simulink model "Stage_3_Multi_ECU_CAN_Network"  (R2025a)
settings: Solver=VariableStepAuto  StartTime=0.0  StopTime=10.0  RelTol=1e-3
libraries: SignalEditorBlockLib x13, canmsglib x8, simulink x1
settings Model: Creator=sitam  LastModifiedBy=sitam

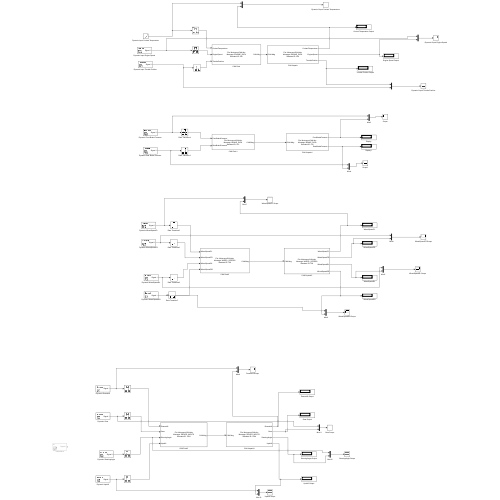
[thumbnail: Simulink's stored preview of the top-level diagram]
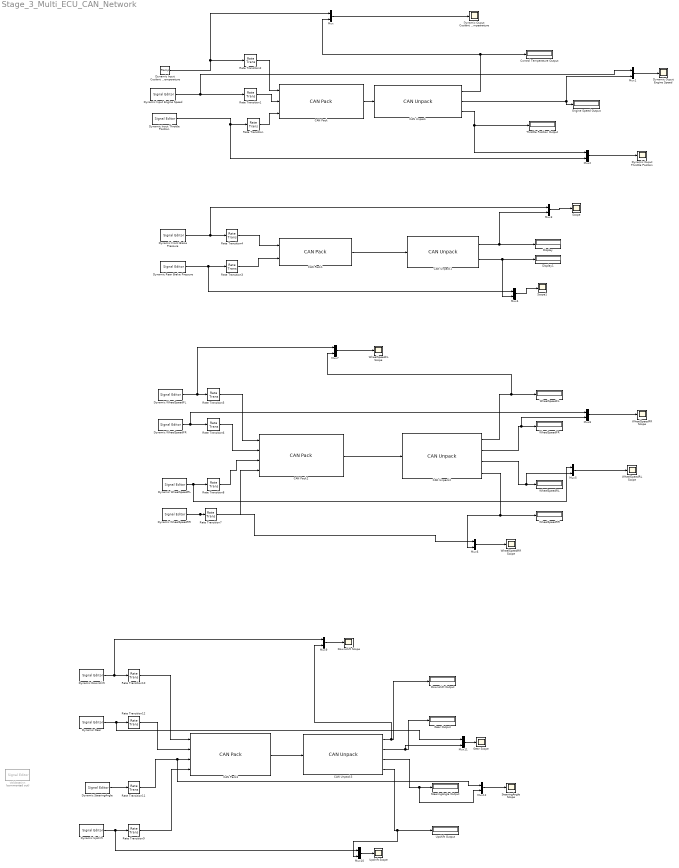
== system Stage_3_Multi_ECU_CAN_Network ==
  CAN Pack : canmsglib/CAN Pack  CANdbFile=C:\Users\sitam\OneDrive\Projects\CAN Bus Project\MotorsportCAN.dbc  MsgList=ENGINE_DATA  MsgName=ENGINE_DATA  MsgIDType=Standard (11-bit identifier)  MsgIdentifier=256  CANIDInput=off  MsgLength=8  Remote=off  ApplyMinMax=off  BusOutput=off  SignalInfo={'CoolantTemperature','24','8','LE','unsigned','Standard','0','1','-40','-40','150';'EngineSpeed','0','16','LE','unsigned','Standard','0','0.25','0','0','15000';'ThrottlePosition','16','8','LE','unsigned','Standard','0','0.4','0','0','100'}
      settings: LibrarySourceBlock=canlib/CAN Pack  DataFormat=CANdb specified signals
  CAN Pack1 : canmsglib/CAN Pack  CANdbFile=C:\Users\sitam\OneDrive\Projects\CAN Bus Project\MotorsportCAN.dbc  MsgList=BRAKE_DATA  MsgName=BRAKE_DATA  MsgIDType=Standard (11-bit identifier)  MsgIdentifier=512  CANIDInput=off  MsgLength=8  Remote=off  ApplyMinMax=off  BusOutput=off  SignalInfo={'FrontBrakePressure','0','16','LE','unsigned','Standard','0','0.01','0','0','200';'RearBrakePressure','16','16','LE','unsigned','Standard','0','0.01','0','0','200'}
      settings: LibrarySourceBlock=canlib/CAN Pack  DataFormat=CANdb specified signals
  CAN Pack2 : canmsglib/CAN Pack  CANdbFile=C:\Users\sitam\OneDrive\Projects\CAN Bus Project\MotorsportCAN.dbc  MsgList=WHEEL_SPEEDS  MsgName=WHEEL_SPEEDS  MsgIDType=Standard (11-bit identifier)  MsgIdentifier=768  CANIDInput=off  MsgLength=8  Remote=off  ApplyMinMax=off  BusOutput=off  SignalInfo={'WheelSpeedFL','0','16','LE','unsigned','Standard','0','0.01','0','0','350';'WheelSpeedFR','16','16','LE','unsigned','Standard','0','0.01','0','0','350';'WheelSpeedRL','32','16','LE','unsigned','Standard','0','0.01','0','0','350';'WheelSpeedRR','48','16','LE','unsigned','Standard','0','0.01','0','0','350'}
      settings: LibrarySourceBlock=canlib/CAN Pack  DataFormat=CANdb specified signals
  CAN Pack3 : canmsglib/CAN Pack  CANdbFile=C:\Users\sitam\OneDrive\Projects\CAN Bus Project\MotorsportCAN.dbc  MsgList=DRIVER_INPUTS  MsgName=DRIVER_INPUTS  MsgIDType=Standard (11-bit identifier)  MsgIdentifier=1024  CANIDInput=off  MsgLength=8  Remote=off  ApplyMinMax=off  BusOutput=off  SignalInfo={'Downshift','25','1','LE','unsigned','Standard','0','1','0','0','1';'Gear','16','3','LE','unsigned','Standard','0','1','0','0','7';'SteeringAngle','0','16','LE','signed','Standard','0','0.1','0','-540','540';'Upshift','24','1','LE','unsigned','Standard','0','1','0','0','1'}
      settings: LibrarySourceBlock=canlib/CAN Pack  DataFormat=CANdb specified signals
  CAN Unpack : canmsglib/CAN Unpack  CANdbFile=C:\Users\sitam\OneDrive\Projects\CAN Bus Project\MotorsportCAN.dbc  MsgList=ENGINE_DATA  MsgName=ENGINE_DATA  MsgIDType=Standard (11-bit identifier)  MsgIdentifier=256  MsgLength=8  SignalInfo={'CoolantTemperature','24','8','LE','unsigned','Standard','0','1','-40','-40','150';'EngineSpeed','0','16','LE','unsigned','Standard','0','0.25','0','0','15000';'ThrottlePosition','16','8','LE','unsigned','Standard','0','0.4','0','0','100'}  IDPort=off  TimestampPort=off  ErrorPort=off  RemotePort=off  LengthPort=off  StatusPort=off  ApplyMinMax=off
      settings: LibrarySourceBlock=canlib/CAN Unpack  DataFormat=CANdb specified signals
  CAN Unpack1 : canmsglib/CAN Unpack  CANdbFile=C:\Users\sitam\OneDrive\Projects\CAN Bus Project\MotorsportCAN.dbc  MsgList=BRAKE_DATA  MsgName=BRAKE_DATA  MsgIDType=Standard (11-bit identifier)  MsgIdentifier=512  MsgLength=8  SignalInfo={'FrontBrakePressure','0','16','LE','unsigned','Standard','0','0.01','0','0','200';'RearBrakePressure','16','16','LE','unsigned','Standard','0','0.01','0','0','200'}  IDPort=off  TimestampPort=off  ErrorPort=off  RemotePort=off  LengthPort=off  StatusPort=off  ApplyMinMax=off
      settings: LibrarySourceBlock=canlib/CAN Unpack  DataFormat=CANdb specified signals
  CAN Unpack2 : canmsglib/CAN Unpack  CANdbFile=C:\Users\sitam\OneDrive\Projects\CAN Bus Project\MotorsportCAN.dbc  MsgList=WHEEL_SPEEDS  MsgName=WHEEL_SPEEDS  MsgIDType=Standard (11-bit identifier)  MsgIdentifier=768  MsgLength=8  SignalInfo={'WheelSpeedFL','0','16','LE','unsigned','Standard','0','0.01','0','0','350';'WheelSpeedFR','16','16','LE','unsigned','Standard','0','0.01','0','0','350';'WheelSpeedRL','32','16','LE','unsigned','Standard','0','0.01','0','0','350';'WheelSpeedRR','48','16','LE','unsigned','Standard','0','0.01','0','0','350'}  IDPort=off  TimestampPort=off  ErrorPort=off  RemotePort=off  LengthPort=off  StatusPort=off  ApplyMinMax=off
      settings: LibrarySourceBlock=canlib/CAN Unpack  DataFormat=CANdb specified signals
  CAN Unpack3 : canmsglib/CAN Unpack  CANdbFile=C:\Users\sitam\OneDrive\Projects\CAN Bus Project\MotorsportCAN.dbc  MsgList=DRIVER_INPUTS  MsgName=DRIVER_INPUTS  MsgIDType=Standard (11-bit identifier)  MsgIdentifier=1024  MsgLength=8  SignalInfo={'Downshift','25','1','LE','unsigned','Standard','0','1','0','0','1';'Gear','16','3','LE','unsigned','Standard','0','1','0','0','7';'SteeringAngle','0','16','LE','signed','Standard','0','0.1','0','-540','540';'Upshift','24','1','LE','unsigned','Standard','0','1','0','0','1'}  IDPort=off  TimestampPort=off  ErrorPort=off  RemotePort=off  LengthPort=off  StatusPort=off  ApplyMinMax=off
      settings: LibrarySourceBlock=canlib/CAN Unpack  DataFormat=CANdb specified signals
  Control Temperature Output : Display
  Display : Display
  Display1 : Display
  Downshift Output : Display
  Downshift Scope : Scope
      settings: ActiveDisplayYMinimum=-1  ActiveDisplayYMaximum=1  DataLoggingVariableName=ScopeData10
  Dynamic Downshift : SignalEditorBlockLib/Signal Editor  FileName=3_downshift.mat  ActiveScenario=Scenario  ActiveSignal=Signal 1  IsBus=off  OutputBusObjectStr=Bus: BusObject  SampleTime=0  ZeroCross=off  OutputAfterFinalValue=Setting to zero  Unit=inherit  PreserveSignalName=on  ApplySigPropsToAllScenarios=on  ApplySigPropsToAllSignals=off  SignalPropertySource=Dialog parameters
  Dynamic Front Brake Pressure : SignalEditorBlockLib/Signal Editor  FileName=3_frontbrake.mat  ActiveScenario=Scenario  ActiveSignal=Signal 1  IsBus=off  OutputBusObjectStr=Bus: BusObject  SampleTime=0  ZeroCross=off  OutputAfterFinalValue=Setting to zero  Unit=inherit  PreserveSignalName=on  ApplySigPropsToAllScenarios=on  ApplySigPropsToAllSignals=off  SignalPropertySource=Dialog parameters
  Dynamic Gear : SignalEditorBlockLib/Signal Editor  FileName=3_gear.mat  ActiveScenario=Scenario  ActiveSignal=Signal 1  IsBus=off  OutputBusObjectStr=Bus: BusObject  SampleTime=0  ZeroCross=off  OutputAfterFinalValue=Setting to zero  Unit=inherit  PreserveSignalName=on  ApplySigPropsToAllScenarios=on  ApplySigPropsToAllSignals=off  SignalPropertySource=Dialog parameters
  Dynamic Input Coolant Temperature : simulink/Sources/Ramp  slope=1  start=0  InitialOutput=85
  Dynamic Input Engine Speed : SignalEditorBlockLib/Signal Editor  FileName=2_2-enginespeed.mat  ActiveScenario=Scenario  ActiveSignal=Signal 1  IsBus=off  OutputBusObjectStr=Bus: BusObject  SampleTime=0  ZeroCross=off  OutputAfterFinalValue=Setting to zero  Unit=inherit  PreserveSignalName=on  ApplySigPropsToAllScenarios=on  ApplySigPropsToAllSignals=off  SignalPropertySource=Dialog parameters
  Dynamic Input Throttle Position : SignalEditorBlockLib/Signal Editor  FileName=2_2-throttlepos.mat  ActiveScenario=Scenario  ActiveSignal=Signal 1  IsBus=off  OutputBusObjectStr=Bus: BusObject  SampleTime=0  ZeroCross=off  OutputAfterFinalValue=Setting to zero  Unit=inherit  PreserveSignalName=on  ApplySigPropsToAllScenarios=on  ApplySigPropsToAllSignals=off  SignalPropertySource=Dialog parameters
  Dynamic Ouput Coolant Tempearature : Scope
      settings: ActiveDisplayYMinimum=83.75  ActiveDisplayYMaximum=96.25
  Dynamic Ouput Engine Speed : Scope
      settings: ActiveDisplayYMinimum=-3441.5893278301937  ActiveDisplayYMaximum=14791.004422169823  DataLoggingVariableName=ScopeData2
  Dynamic Ouput Throttle Position : Scope
      settings: ActiveDisplayYMinimum=-6.6313525458429439  ActiveDisplayYMaximum=101.34834727059156
  Dynamic Rear Brake Pressure : SignalEditorBlockLib/Signal Editor  FileName=3_rearbrake.mat  ActiveScenario=Scenario  ActiveSignal=Signal 1  IsBus=off  OutputBusObjectStr=Bus: BusObject  SampleTime=0  ZeroCross=off  OutputAfterFinalValue=Setting to zero  Unit=inherit  PreserveSignalName=on  ApplySigPropsToAllScenarios=on  ApplySigPropsToAllSignals=off  SignalPropertySource=Dialog parameters
  Dynamic SteeringAngle : SignalEditorBlockLib/Signal Editor  FileName=3_steeringangle.mat  ActiveScenario=Scenario  ActiveSignal=Signal 1  IsBus=off  OutputBusObjectStr=Bus: BusObject  SampleTime=0  ZeroCross=off  OutputAfterFinalValue=Setting to zero  Unit=inherit  PreserveSignalName=on  ApplySigPropsToAllScenarios=on  ApplySigPropsToAllSignals=off  SignalPropertySource=Dialog parameters
  Dynamic Upshift : SignalEditorBlockLib/Signal Editor  FileName=3_upshift.mat  ActiveScenario=Scenario  ActiveSignal=Signal 1  IsBus=off  OutputBusObjectStr=Bus: BusObject  SampleTime=0  ZeroCross=off  OutputAfterFinalValue=Setting to zero  Unit=inherit  PreserveSignalName=on  ApplySigPropsToAllScenarios=on  ApplySigPropsToAllSignals=off  SignalPropertySource=Dialog parameters
  Dynamic WheelSpeedFL : SignalEditorBlockLib/Signal Editor  FileName=3_WheelSpeedFL.mat  ActiveScenario=Scenario  ActiveSignal=Signal 1  IsBus=off  OutputBusObjectStr=Bus: BusObject  SampleTime=0  ZeroCross=off  OutputAfterFinalValue=Setting to zero  Unit=inherit  PreserveSignalName=on  ApplySigPropsToAllScenarios=on  ApplySigPropsToAllSignals=off  SignalPropertySource=Dialog parameters
  Dynamic WheelSpeedFR : SignalEditorBlockLib/Signal Editor  FileName=3_WheelSpeedFR.mat  ActiveScenario=Scenario  ActiveSignal=Signal 1  IsBus=off  OutputBusObjectStr=Bus: BusObject  SampleTime=0  ZeroCross=off  OutputAfterFinalValue=Setting to zero  Unit=inherit  PreserveSignalName=on  ApplySigPropsToAllScenarios=on  ApplySigPropsToAllSignals=off  SignalPropertySource=Dialog parameters
  Dynamic WheelSpeedRL : SignalEditorBlockLib/Signal Editor  FileName=3_WheelSpeedRL.mat  ActiveScenario=Scenario  ActiveSignal=Signal 1  IsBus=off  OutputBusObjectStr=Bus: BusObject  SampleTime=0  ZeroCross=off  OutputAfterFinalValue=Setting to zero  Unit=inherit  PreserveSignalName=on  ApplySigPropsToAllScenarios=on  ApplySigPropsToAllSignals=off  SignalPropertySource=Dialog parameters
  Dynamic WheelSpeedRR : SignalEditorBlockLib/Signal Editor  FileName=3_WheelSpeedRR.mat  ActiveScenario=Scenario  ActiveSignal=Signal 1  IsBus=off  OutputBusObjectStr=Bus: BusObject  SampleTime=0  ZeroCross=off  OutputAfterFinalValue=Setting to zero  Unit=inherit  PreserveSignalName=on  ApplySigPropsToAllScenarios=on  ApplySigPropsToAllSignals=off  SignalPropertySource=Dialog parameters
  Engine Speed Output : Display
  Gear Output : Display
  Gear Scope : Scope
      settings: ActiveDisplayYMinimum=1  ActiveDisplayYMaximum=3  DataLoggingVariableName=ScopeData12
  Mux{,1..12} (13 alike) : Mux  Inputs=2
  Rate Transition{,1..4} (5 alike) : RateTransition  OutPortSampleTime=0.01
  Rate Transition{9..12} (4 alike) : RateTransition  OutPortSampleTime=0.02
  Rate Transition{5..8} (4 alike) : RateTransition  OutPortSampleTime=0.005
  Scope : Scope
      settings: ActiveDisplayYMinimum=-14.999999999999996  ActiveDisplayYMaximum=135  DataLoggingVariableName=ScopeData3
  Scope1 : Scope
      settings: ActiveDisplayYMinimum=-9.3749999999999982  ActiveDisplayYMaximum=84.375  DataLoggingVariableName=ScopeData4
  SteeringAngle Output : Display
  SteeringAngle Scope : Scope
      settings: ActiveDisplayYMinimum=-5.9620958433066278  ActiveDisplayYMaximum=209.99730378956232  DataLoggingVariableName=ScopeData9
  Throttle Position Output : Display
  Upshift Output : Display
  Upshift Scope : Scope
      settings: ActiveDisplayYMinimum=-1  ActiveDisplayYMaximum=1  DataLoggingVariableName=ScopeData11
  Validatation : SignalEditorBlockLib/Signal Editor  Commented=on  FileName=alidate.mat  ActiveScenario=Scenario  ActiveSignal=Signal 1  IsBus=off  OutputBusObjectStr=Bus: BusObject  SampleTime=0  ZeroCross=off  OutputAfterFinalValue=Setting to zero  Unit=inherit  PreserveSignalName=on  ApplySigPropsToAllScenarios=on  ApplySigPropsToAllSignals=off  SignalPropertySource=Dialog parameters
  WheelSpeedFL : Display
  WheelSpeedFL Scope : Scope
      settings: ActiveDisplayYMinimum=-1  ActiveDisplayYMaximum=1  DataLoggingVariableName=ScopeData6
  WheelSpeedFR : Display
  WheelSpeedFR Scope : Scope
      settings: ActiveDisplayYMinimum=-1  ActiveDisplayYMaximum=1  DataLoggingVariableName=ScopeData8
  WheelSpeedRL : Display
  WheelSpeedRL Scope : Scope
      settings: ActiveDisplayYMinimum=-1  ActiveDisplayYMaximum=1  DataLoggingVariableName=ScopeData7
  WheelSpeedRR : Display
  WheelSpeedRR Scope : Scope
      settings: ActiveDisplayYMinimum=-1  ActiveDisplayYMaximum=1  DataLoggingVariableName=ScopeData5
  wires:
  CAN Pack/1 -> CAN Unpack/1
  CAN Unpack/2 -> Engine Speed Output/1, Mux1/2
  CAN Unpack/1 -> Mux/2, Control Temperature Output/1
  CAN Unpack/3 -> Mux2/1, Throttle Position Output/1
  Dynamic Input Coolant Temperature/1 -> Mux/1, Rate Transition2/1
  Dynamic Input Engine Speed/1 -> Mux1/1, Rate Transition1/1
  Dynamic Input Throttle Position/1 -> Mux2/2, Rate Transition/1
  Mux/1 -> Dynamic Ouput Coolant Tempearature/1
  Mux1/1 -> Dynamic Ouput Engine Speed/1
  Mux2/1 -> Dynamic Ouput Throttle Position/1
  Rate Transition2/1 -> CAN Pack/1
  Rate Transition1/1 -> CAN Pack/2
  Rate Transition/1 -> CAN Pack/3
  CAN Pack1/1 -> CAN Unpack1/1
  Rate Transition4/1 -> CAN Pack1/1
  Rate Transition3/1 -> CAN Pack1/2
  Dynamic Front Brake Pressure/1 -> Mux3/1, Rate Transition4/1
  Dynamic Rear Brake Pressure/1 -> Mux4/1, Rate Transition3/1
  CAN Unpack1/1 -> Mux3/2, Display/1
  CAN Unpack1/2 -> Mux4/2, Display1/1
  Mux4/1 -> Scope1/1
  Mux3/1 -> Scope/1
  CAN Pack2/1 -> CAN Unpack2/1
  CAN Unpack2/4 -> WheelSpeedRR/1, Mux6/2
  CAN Unpack2/3 -> Mux5/2, WheelSpeedRL/1
  CAN Unpack2/2 -> Mux8/2, WheelSpeedFR/1
  CAN Unpack2/1 -> Mux7/2, WheelSpeedFL/1
  Rate Transition5/1 -> CAN Pack2/1
  Rate Transition6/1 -> CAN Pack2/2
  Rate Transition8/1 -> CAN Pack2/3
  Rate Transition7/1 -> CAN Pack2/4
  Dynamic WheelSpeedFR/1 -> Mux8/1, Rate Transition6/1
  Dynamic WheelSpeedRL/1 -> Mux5/1, Rate Transition8/1
  Dynamic WheelSpeedFL/1 -> Mux7/1, Rate Transition5/1
  Mux7/1 -> WheelSpeedFL Scope/1
  Mux8/1 -> WheelSpeedFR Scope/1
  Mux5/1 -> WheelSpeedRL Scope/1
  Mux6/1 -> WheelSpeedRR Scope/1
  Dynamic WheelSpeedRR/1 -> Mux6/1, Rate Transition7/1
  CAN Pack3/1 -> CAN Unpack3/1
  CAN Unpack3/1 -> Mux9/2, Downshift Output/1
  CAN Unpack3/2 -> Mux11/2, Gear Output/1
  CAN Unpack3/3 -> Mux12/2, SteeringAngle Output/1
  CAN Unpack3/4 -> Mux10/2, Upshift Output/1
  Rate Transition10/1 -> CAN Pack3/1
  Rate Transition12/1 -> CAN Pack3/2
  Rate Transition11/1 -> Mux12/1, CAN Pack3/3
  Rate Transition9/1 -> CAN Pack3/4
  Dynamic Downshift/1 -> Mux9/1, Rate Transition10/1
  Dynamic Gear/1 -> Mux11/1, Rate Transition12/1
  Dynamic Upshift/1 -> Mux10/1, Rate Transition9/1
  Mux9/1 -> Downshift Scope/1
  Mux11/1 -> Gear Scope/1
  Mux12/1 -> SteeringAngle Scope/1
  Mux10/1 -> Upshift Scope/1
  Dynamic SteeringAngle/1 -> Rate Transition11/1
